simulink model "BD_CONV2"  (Simulink 4.1.1)
settings: Solver=ode1  SolverMode=SingleTasking  StartTime=0.0  StopTime=max(cyc_mph(:,1))  FixedStep=1  MaxStep=1  RelTol=1e-3  AbsTol=1e-3
undefined symbols (not defined in the file): cyc_mph, ess_on, ex_calc, fc_ct_trq, fc_emis, fc_inertia, fc_map_spd, fc_max_trq, fc_spd_scale, fc_trq_scale, fd_inertia, fd_loss, fd_ratio, gb_dnshift_load, gb_dnshift_spd, gb_gears_num, gb_inertia, gb_num_init, gb_ratio, gb_shift_delay, gb_spd_scale, gb_trq_scale, gb_upshift_load, gb_upshift_spd, logFlag, tx_eff_map, tx_map_spd, tx_map_trq, vc_clutch_bool, vc_idle_bool, vc_idle_spd, vc_key_on, vc_launch_spd, veh_air_density, veh_CD, veh_FA, veh_gravity, veh_mass, wh_axle_loss_mass, wh_axle_loss_trq, wh_front_active_bool, wh_inertia, wh_max_front_brake_force, wh_max_rear_brake_force, wh_radius, wh_rear_active_bool, wh_slip, wh_slip_force_coeff
libraries: lib_wheel2 x12, lib_drive_cycle2 x2, lib_accessory2 x2, lib_etc x2, lib_interactive x1, lib_exhaust x1, lib_fuel_converter3 x1, lib_help x1
(part 1 of 11)
settings Model: ExecutionOrder=on  LastModifiedBy=mokeefe  SaveTime=off  SaveOutput=off  LimitDataPoints=off  UnconnectedLineMsg=none  RTWTemplateMakefile=grt_vc.tmf  ExtModeTrigMode=oneshot  ExtModeArmWhenConnect=off
settings Model: ModifiedComment=|
  | mokeefe -- Thu Apr 18 07:47:12 2002 -- Version 1.98
  | saving the model:
  | o "without the model browser open"
  | o with only top-level screen visible
  | o and with "fit to view" enabled
settings Model: ModifiedHistory=|
  | mokeefe -- Thu Apr 18 07:47:12 2002 -- Version 1.98
  | saving the model:
  | o "without the model browser open"
  | o with only top-level screen visible
  | o and with "fit to view" enabled
  | 
  | mokeefe -- Thu Apr 18 07:46:46 2002 -- Version 1.97
  | saving the model:
  | o "without the model browser open"
  | o with only top-level screen visible
  | o and with "fit to view" enabled
  | 
  | mokeefe -- Thu Apr 18 07:37:24 2002 -- Version 1.96
  | saving the model
  | "without the model browser open"
  | with only top-level screen visible
  | and with "fit to view" enabled
  | 
  | abrooker -- Fri Apr 12 08:11:12 2002 -- Version 1.95
  | 
  | 
  | abrooker -- Fri Apr 12 08:02:30 2002 -- Version 1.94
  | 
  | 
  | abrooker -- Fri Apr 12 08:02:26 2002 -- Version 1.93
  | 
  | 
  | abrooker -- Fri Apr 12 07:59:19 2002 -- Version 1.92
  | 
  | 
  | abrooker -- Fri Apr 12 07:49:13 2002 -- Version 1.91
  | 
  | 
  | mokeefe -- Fri Mar 29 15:46:36 2002 -- Version 1.90
  | 
  | 
  | mokeefe -- Wed Mar 06 11:56:56 2002 -- Version 1.89
  | 
  | 
  | mokeefe -- Wed Mar 06 11:56:30 2002 -- Version 1.88
  | changed the acc_on flag in mechanical accessory loads
  | 
  | mokeefe -- Tue Mar 05 14:28:10 2002 -- Version 1.87
  | 
  | 
  | mokeefe -- Mon Mar 04 14:59:21 2002 -- Version 1.86
  | changed engine_on to key_on in Mechanical Accessory Loads <acc>
  | 
  | mokeefe -- Mon Mar 04 07:29:42 2002 -- Version 1.85
  | 
  | 
  | mokeefe -- Mon Mar 04 07:29:35 2002 -- Version 1.84
  | 
  | 
  | mokeefe -- Fri Mar 01 16:40:39 2002 -- Version 1.83
  | 
  | 
  | mokeefe -- Fri Mar 01 15:08:54 2002 -- Version 1.82
  | 
  | 
  | mokeefe -- Fri Mar 01 12:12:36 2002 -- Version 1.81
  | 
  | 
  | mokeefe -- Fri Mar 01 11:41:50 2002 -- Version 1.80
  | 
  | 
  | mokeefe -- Fri Mar 01 11:21:25 2002 -- Version 1.79
  | 
  | 
  | mokeefe -- Fri Mar 01 10:51:16 2002 -- Version 1.78
  | 
  | 
  | mokeefe -- Fri Mar 01 10:28:03 2002 -- Version 1.77
  | 
  | 
  | mokeefe -- Fri Mar 01 10:27:49 2002 -- Version 1.76
  | 
  | 
  | mokeefe -- Fri Mar 01 10:27:36 2002 -- Version 1.75
  | 
  | 
  | mokeefe -- Thu Feb 28 08:54:13 2002 -- Version 1.74
  | 
  | 
  | mokeefe -- Thu Feb 28 08:41:46 2002 -- Version 1.73
  | 
  | 
  | mokeefe -- Thu Feb 28 08:40:29 2002 -- Version 1.72
  | 
  | 
  | mokeefe -- Thu Feb 28 08:37:03 2002 -- Version 1.71
  | 
  | 
  | mokeefe -- Thu Feb 28 08:29:13 2002 -- Version 1.70
  | changing the mechanical auxiliary loads block to be more simplistic
  | 
  | mokeefe -- Wed Feb 27 14:39:18 2002 -- Version 1.69
  | 
  | 
  | mokeefe -- Wed Feb 27 14:38:57 2002 -- Version 1.68
  | 
  | 
  | mokeefe -- Wed Feb 27 14:16:01 2002 -- Version 1.67
  | changing to Mechanical Accessory Loads v2 <acc> from lib_accessory
  | 
  | mokeefe -- Wed Feb 27 14:14:56 2002 -- Version 1.66
  | 
  | 
  | mokeefe -- Tue Feb 26 10:43:51 2002 -- Version 1.65
  | changing the way that the auxiliary loads are calculated and logged to workspace. Electrical loads run on a conventional powertrain are assumed to have a mechanical to electrical efficiency penalty but are translated and added as mechanical loads
  | 
  | mokeefe -- Tue Feb 26 10:36:09 2002 -- Version 1.64
  | 
  | 
  | mokeefe -- Tue Feb 26 09:51:22 2002 -- Version 1.63
  | changed the condition for whether electrical loads are accounted in auxiliary loads block (Mechanical Accessory Loads <acc>) to be not(ess_on)
  | 
  | mokeefe -- Mon Feb 25 15:04:18 2002 -- Version 1.62
  | 
  | 
  | mokeefe -- Mon Feb 25 14:59:54 2002 -- Version 1.61
  | 
  | 
  | mokeefe -- Mon Feb 25 14:24:21 2002 -- Version 1.60
  | 
  | 
  | mokeefe -- Fri Feb 15 11:53:40 2002 -- Version 1.59
  | added and tested  Mechanical Accessory Loads <acc> block
  | 
  | mokeefe -- Thu Feb 14 17:56:13 2002 -- Version 1.58
  | 
  | 
  | mokeefe -- Thu Feb 14 17:21:52 2002 -- Version 1.57
  | 
  | 
  | mokeefe -- Thu Feb 14 17:05:06 2002 -- Version 1.56
  | updated with Mechanical Accessory Loads <acc> block
  | 
  | mokeefe -- Thu Feb 14 16:31:11 2002 -- Version 1.55
  | 
  | 
  | mokeefe -- Thu Feb 14 16:04:04 2002 -- Version 1.54
  | added Mechanical Auxiliary Loads (acc) block
  | 
  | mokeefe -- Thu Feb 14 10:48:35 2002 -- Version 1.53
  | 
  | 
  | mokeefe -- Thu Feb 14 10:41:17 2002 -- Version 1.52
  | 
  | 
  | mokeefe -- Thu Feb 14 10:24:42 2002 -- Version 1.51
  | 
  | 
  | mokeefe -- Thu Feb 14 09:59:11 2002 -- Version 1.50
  | testing
  | 
  | 
  | ssprik -- Fri Feb 09 15:14:35 2001 -- Version 1.49
  | changed foregrounds to black colors

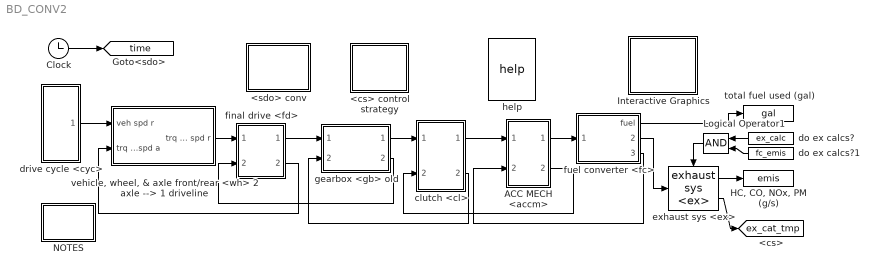
== system BD_CONV2 ==
  <cs> control strategy : Subsystem
      settings: RTWFcnNameOpts=Auto  RTWFileNameOpts=Auto
      mask Display: image(imread('bdi_cs.jpg'))
  <sdo> conv : Subsystem
      settings: RTWFcnNameOpts=Auto  RTWFileNameOpts=Auto
      mask Display: image(imread('bdi_sdo.jpg'))
  ACC MECH <accm> : Subsystem  AncestorBlock=lib_accessory2/ACC MECH <accm>  mask(Stand-Alone Mechanical Accessory Mask){generalName='acc', logPick=Log, initFileName={}, modCell={}, imgFileName='bdi_acc_pic.bmp', DEBUG=OFF}
      mask prompts: generalName "General Name of this Component [char]"; logPick "Log Variables to Workspace?"; initFileName "Initialization File(s) [cell array of char]"; modCell "Modification Cell [2 column cell array of param and val]"; imgFileName "Icon image file name [char--evaluated]"
      mask init:
      | % initialization via m-file script
      | advSACompMaskInit;
      settings: RTWFcnNameOpts=Auto  RTWFileNameOpts=Auto
      mask StyleString: edit,popup(Don't Log|Log),edit,edit,edit,popup(ON|OFF)
      mask Display: image(imread(imgFileName))
  Clock : Clock
      settings: DisplayTime=off  Decimation=10
  "HC, CO, NOx, PM (g/s)" : ToWorkspace  VariableName=emis  SampleTime=0  SaveFormat=Array
  Interactive Graphics : Subsystem  BlockChoice=off
      settings: AttributesFormatString=%<BlockChoice>  TemplateBlock=lib_interactive/Interactive Graphics  MemberBlocks=off,on  RTWFcnNameOpts=Auto  RTWFileNameOpts=Auto
  Logical Operator1 : Logic  Orientation=left  Operator=AND  Inputs=2
  NOTES : Subsystem
      settings: RTWFcnNameOpts=Auto  RTWFileNameOpts=Auto
      mask Display: disp('Version &\nCopyright')
  clutch <cl> : Subsystem  AncestorBlock=lib_transmission2/clutch <cl>  mask(Stand-Alone Clutch Mask){generalName='cl', logPick=Log, initFileName={}, modCell={}, imgFileName='bdi_cl.jpg', slip_spd=vc_launch_spd, maxtrq=max(fc_max_trq)*fc_trq_scale, DEBUG=OFF}
      mask prompts: generalName "General Name of this Component [char--evaluated]"; logPick "Log Variables to Workspace?"; initFileName "Initialization File(s) [cell array of char]"; modCell "Modification Cell [2 column cell array of param and val]"; imgFileName "Icon image file name [char--evaluated]"; slip_spd "Input shaft speed when clutch slips (rad/s):"; maxtrq "Maximum torque clutch can transmit:"
      mask help: Clutch for use with ADVISOR 2
      mask init:
      | % initialization via m-file script
      | advSACompMaskInit;
      settings: RTWFcnNameOpts=Auto  RTWFileNameOpts=Auto
      mask Help:
      | First input is req'd clutch output torque and speed, muxed together.
      | Second input is clutch state, with 1 => disengaged, 2 => slipping, and 3=> engaged.
      | Third input is available clutch input torque and limited clutch input speed.
      | First output is req'd clutch input torque and speed, muxed together.
      | Second output is available clutch output torque and limited clutch output speed.
      | The logic implemented by this block is as follows:
      |           IF (clutch is disengaged) THEN (req'd input torque=0), (req'd input speed=req'd output speed (the engine control is responsible for computing correct engine spin-down speed)), (avail. output torque=0), (limited output speed=req'd output speed)
      |           IF (clutch is slipping) THEN (req'd input torque=req'd output torque), (req'd input speed=user-defined slip speed), (avail. output torque=avail. input torque), (limited output speed=req'd output speed)
      |           IF (clutch is engaged) THEN (req'd input torque=req'd output torque), (req'd input speed=req'd output speed), (avail. output torque=avail. input torque), (limited output speed=limited input speed)
      | 
      | The clutch will transmit no more than its maximum torque as driving or braking torque.
      mask StyleString: edit,popup(Don't Log|Log),edit,edit,edit,edit,edit,popup(ON|OFF)
      mask Display: image(imread(imgFileName))
  do ex calcs? : Constant  Orientation=left  Value=ex_calc
  do ex calcs?1 : Constant  Orientation=left  Value=fc_emis
  drive cycle <cyc> : Subsystem  AncestorBlock=lib_drive_cycle2/drive cycle <cyc>  mask(Stand-Alone Drive Cycle Mask){generalName='cyc', logPick=Log, initFileName={}, modCell={}, imgFileName='bdi_cyc.jpg', DEBUG=OFF, veh_mass=veh_mass}
      mask prompts: generalName "General Name of this Component [char]"; logPick "Log Variables to Workspace?"; initFileName "Initialization File(s) [cell array of char]"; modCell "Modification Cell [2 column cell array of param and val]"; imgFileName "Icon image file name [char--evaluated]"; veh_mass "Vehicle Mass (kg)"
      mask init:
      | % initialization via m-file script
      | advSACompMaskInit;
      settings: RTWFcnNameOpts=Auto  RTWFileNameOpts=Auto
      mask StyleString: edit,popup(Don't Log|Log),edit,edit,edit,popup(ON|OFF),edit
      mask Display: image(imread(imgFileName))
  exhaust sys <ex> : lib_exhaust/exhaust sys <ex>
  final drive <fd> : Subsystem  AncestorBlock=lib_transmission2/final drive <fd>  mask(Stand-Alone Final Drive Mask){generalName='fd', logPick=Log, initFileName={}, modCell={}, imgFileName='bdi_fd.jpg', DEBUG=OFF}
      mask prompts: generalName "General Name of this Component [char]"; logPick "Log Variables to Workspace?"; initFileName "Initialization File(s) [cell array of char]"; modCell "Modification Cell [2 column cell array of param and val]"; imgFileName "Icon image file name [char--evaluated]"
      mask init:
      | % initialization via m-file script
      | advSACompMaskInit;
      settings: RTWFcnNameOpts=Auto  RTWFileNameOpts=Auto
      mask StyleString: edit,popup(Don't Log|Log),edit,edit,edit,popup(ON|OFF)
      mask Display: image(imread(imgFileName))
  fuel converter <fc> : Subsystem  AncestorBlock=lib_fuel_converter3/fuel converter <fc>  mask(Stand-Alone IC ENGINE Mask){generalName='fc', logPick=Log, initFileName={}, modCell={}, imgFileName='bdi_fc.jpg', DEBUG=OFF}
      mask prompts: generalName "General Name of this Component [char]"; logPick "Log Variables to Workspace?"; initFileName "Initialization File(s) [cell array of char]"; modCell "Modification Cell [2 column cell array of param and val]"; imgFileName "Icon image file name [char--evaluated]"
      mask init:
      | % initialization via m-file script
      | advSACompMaskInit;
      settings: RTWFcnNameOpts=Auto  RTWFileNameOpts=Auto
      mask StyleString: edit,popup(Don't Log|Log),edit,edit,edit,popup(ON|OFF)
      mask Display: image(imread(imgFileName))
  gearbox <gb> old : Subsystem  AncestorBlock=lib_transmission2/gearbox <gb> old  mask(Stand-Alone Gearbox Mask){generalName='gb', logPick=Log, initFileName={}, modCell={}, imgFileName='bdi_gb.jpg', DEBUG=OFF}
      mask prompts: generalName "General Name of this Component [char]"; logPick "Log Variables to Workspace?"; initFileName "Initialization File(s) [cell array of char]"; modCell "Modification Cell [2 column cell array of param and val]"; imgFileName "Icon image file name [char--evaluated]"
      mask init:
      | % initialization via m-file script
      | advSACompMaskInit;
      settings: RTWFcnNameOpts=Auto  RTWFileNameOpts=Auto
      mask StyleString: edit,popup(Don't Log|Log),edit,edit,edit,popup(ON|OFF)
      mask Display: image(imread(imgFileName))
  help : lib_help/help
  total fuel used (gal) : ToWorkspace  VariableName=gal  SampleTime=0  SaveFormat=Array
  "vehicle, wheel, & axle front/rear <wh> 2 axle --> 1 driveline" : Subsystem  AncestorBlock=|  mask(Stand-Alone Vehicle, Wheel, & Axle Mask){generalName='veh', generalName01='wh', logPick=Log, initFileName={}, modCell={}, imgFileName='bdi_wh&veh.jpg', DEBUG=OFF}
      | lib_wheel2/vehicle, wheel, & axle
      | front//rear <wh>
      | 2 axle --> 1 driveline
      mask prompts: generalName "General Name of Vehicle Component [char]"; generalName01 "General Name of Wheel Component [char]"; logPick "Log Variables to Workspace?"; initFileName "Initialization File(s) for VEH and WH [cell array of char]"; modCell "Modification Cell [2 column cell array of param and val]"; imgFileName "Icon image file name [char--evaluated]"
      mask init:
      | % initialization via m-file script
      | advSACompMaskInit;
      settings: RTWFcnNameOpts=Auto  RTWFileNameOpts=Auto
      mask StyleString: edit,edit,popup(Don't Log|Log),edit,edit,edit,popup(ON|OFF)
      mask Display: image(imread(imgFileName))
  tag scope: ex_cat_tmp=global, time=global
  wires:
  Clock/1 -> [time]
  final drive <fd>/1("torque and speed req'd at input side of final drive (Nm), (rad/s)") -> gearbox <gb> old/1("torque and speed req'd at output side of gearbox (Nm), (rad/s)")
  gearbox <gb> old/2("torque and speed avail. at output side of gearbox (Nm), (rad/s)") -> final drive <fd>/2("torque and speed avail. at input side of final drive (Nm), (rad/s)")
  drive cycle <cyc>/1(req'd vehicle speed (m/s)) -> "vehicle, wheel, & axle front/rear <wh> 2 axle --> 1 driveline"/1(veh spd r)
  gearbox <gb> old/1("torque and speed req'd at input side of gearbox (Nm), (rad/s)") -> clutch <cl>/1(T & w output requested)
  clutch <cl>/2(T & w output achieved) -> gearbox <gb> old/2("torque and speed avail. at input side of gearbox (Nm), (rad/s)")
  fuel converter <fc>/2(engine out emissions) -> exhaust sys <ex>/1
  fuel converter <fc>/1(fuel) -> total fuel used (gal)/1
  exhaust sys <ex>/1 -> "HC, CO, NOx, PM (g/s)"/1
  Logical Operator1/1 -> exhaust sys <ex>/Enable
  do ex calcs?/1 -> Logical Operator1/1
  do ex calcs?1/1 -> Logical Operator1/2
  exhaust sys <ex>/2 -> [ex_cat_tmp]
  clutch <cl>/1(T & w input request) -> ACC MECH <accm>/1(trq and spd out requested)
  fuel converter <fc>/3(trq and spd out achieved) -> ACC MECH <accm>/2(trq and spd in achieved)
  "vehicle, wheel, & axle front/rear <wh> 2 axle --> 1 driveline"/1(trq & spd r) -> final drive <fd>/1("torque and speed req'd at output side of final drive (Nm), (rad/s)")
  final drive <fd>/2("torque and speed avail. at output side of final drive (Nm), (rad/s)") -> "vehicle, wheel, & axle front/rear <wh> 2 axle --> 1 driveline"/2(trq & spd a)
  ACC MECH <accm>/1(trq and spd in  requested) -> fuel converter <fc>/1(trq and spd out requested)
  ACC MECH <accm>/2("trq and spd out achieved ") -> clutch <cl>/2(T & w input achieved)

== system BD_CONV2/<cs> control strategy ==
  Clutch Control : Subsystem
      settings: RTWFcnNameOpts=Auto  RTWFileNameOpts=Auto
  Drive Cycle : Subsystem
      settings: RTWFcnNameOpts=Auto  RTWFileNameOpts=Auto
  Fuel Converter Control conventional ic engine : Subsystem
      settings: RTWFcnNameOpts=Auto  RTWFileNameOpts=Auto
  Gearbox Control manual shift logic : Subsystem
      settings: RTWFcnNameOpts=Auto  RTWFileNameOpts=Auto
  Mechanical Accessories : Subsystem
      settings: RTWFcnNameOpts=Auto  RTWFileNameOpts=Auto
  Wheel Control : Subsystem
      settings: RTWFcnNameOpts=Auto  RTWFileNameOpts=Auto

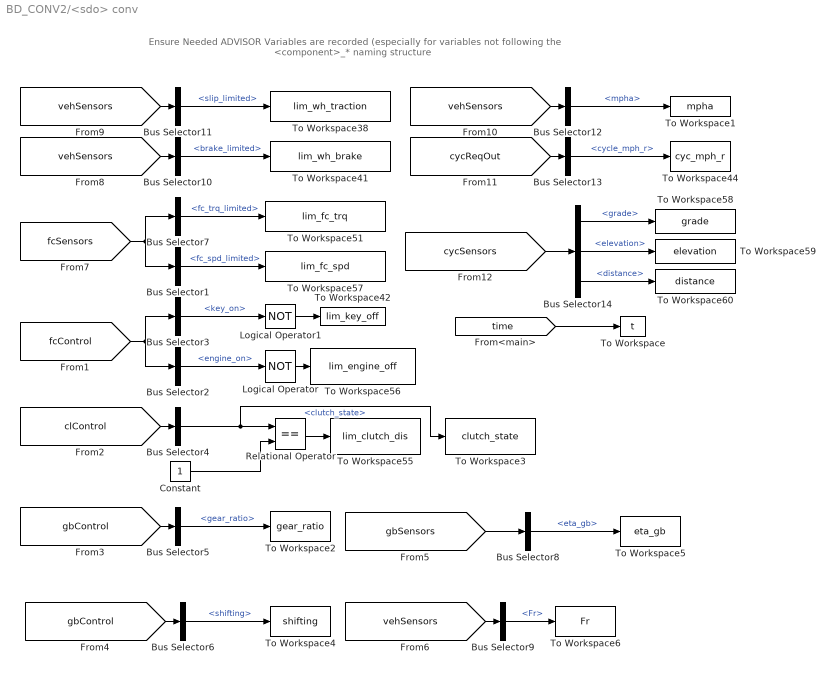
== system BD_CONV2/<sdo> conv ==
  note: Ensure Needed ADVISOR Variables are recorded
      | (especially for variables not following the <component>_* naming structure
  Bus Selector1 : BusSelector  OutputSignals=fc_spd_limited  MuxedOutput=off
  Bus Selector10 : BusSelector  OutputSignals=brake_limited  MuxedOutput=off
  Bus Selector11 : BusSelector  OutputSignals=slip_limited  MuxedOutput=off
  Bus Selector12 : BusSelector  OutputSignals=mpha  MuxedOutput=off
  Bus Selector13 : BusSelector  OutputSignals=cycle_mph_r  MuxedOutput=off
  Bus Selector14 : BusSelector  OutputSignals=grade,elevation,distance  MuxedOutput=off
  Bus Selector2 : BusSelector  OutputSignals=engine_on  MuxedOutput=off
  Bus Selector3 : BusSelector  OutputSignals=key_on  MuxedOutput=off
  Bus Selector4 : BusSelector  OutputSignals=clutch_state  MuxedOutput=off
  Bus Selector5 : BusSelector  OutputSignals=gear_ratio  MuxedOutput=off
  Bus Selector6 : BusSelector  OutputSignals=shifting  MuxedOutput=off
  Bus Selector7 : BusSelector  OutputSignals=fc_trq_limited  MuxedOutput=off
  Bus Selector8 : BusSelector  OutputSignals=eta_gb  MuxedOutput=off
  Bus Selector9 : BusSelector  OutputSignals=Fr  MuxedOutput=off
  Constant : Constant  Value=1
  Logical Operator : Logic  Operator=NOT  Inputs=1
  Logical Operator1 : Logic  Operator=NOT  Inputs=1
  Relational Operator : RelationalOperator  Operator===
  To Workspace : ToWorkspace  VariableName=t  SampleTime=0  SaveFormat=Array
  To Workspace1 : ToWorkspace  VariableName=mpha  SampleTime=-1  SaveFormat=Array
  To Workspace2 : ToWorkspace  VariableName=gear_ratio  SampleTime=-1  SaveFormat=Array
  To Workspace3 : ToWorkspace  VariableName=clutch_state  SampleTime=-1  SaveFormat=Array
  To Workspace38 : ToWorkspace  VariableName=lim_wh_traction  SampleTime=-1  SaveFormat=Array
  To Workspace4 : ToWorkspace  VariableName=shifting  SampleTime=-1  SaveFormat=Array
  To Workspace41 : ToWorkspace  VariableName=lim_wh_brake  SampleTime=-1  SaveFormat=Array
  To Workspace42 : ToWorkspace  VariableName=lim_key_off  SampleTime=-1  SaveFormat=Array
  To Workspace44 : ToWorkspace  VariableName=cyc_mph_r  SampleTime=-1  SaveFormat=Array
  To Workspace5 : ToWorkspace  VariableName=eta_gb  SampleTime=-1  SaveFormat=Array
  To Workspace51 : ToWorkspace  VariableName=lim_fc_trq  SampleTime=-1  SaveFormat=Array
  To Workspace55 : ToWorkspace  VariableName=lim_clutch_dis  SampleTime=-1  SaveFormat=Array
  To Workspace56 : ToWorkspace  VariableName=lim_engine_off  SampleTime=-1  SaveFormat=Array
  To Workspace57 : ToWorkspace  VariableName=lim_fc_spd  SampleTime=-1  SaveFormat=Array
  To Workspace58 : ToWorkspace  VariableName=grade  SampleTime=-1  SaveFormat=Array
  To Workspace59 : ToWorkspace  VariableName=elevation  SampleTime=-1  SaveFormat=Array
  To Workspace6 : ToWorkspace  VariableName=Fr  SampleTime=-1  SaveFormat=Array
  To Workspace60 : ToWorkspace  VariableName=distance  SampleTime=-1  SaveFormat=Array
  wires:
  [time] -> To Workspace/1
  Logical Operator/1 -> To Workspace56/1
  Constant/1 -> Relational Operator/2
  Relational Operator/1 -> To Workspace55/1
  Bus Selector14/3 -> To Workspace60/1  "<distance>"
  Bus Selector14/2 -> To Workspace59/1  "<elevation>"
  Bus Selector14/1 -> To Workspace58/1  "<grade>"
  Logical Operator1/1 -> To Workspace42/1
  [fcSensors] -> Bus Selector7/1, Bus Selector1/1
  Bus Selector7/1 -> To Workspace51/1  "<fc_trq_limited>"
  Bus Selector1/1 -> To Workspace57/1  "<fc_spd_limited>"
  [fcControl] -> Bus Selector3/1, Bus Selector2/1
  Bus Selector2/1 -> Logical Operator/1  "<engine_on>"
  Bus Selector3/1 -> Logical Operator1/1  "<key_on>"
  [clControl] -> Bus Selector4/1
  Bus Selector4/1 -> Relational Operator/1, To Workspace3/1  "<clutch_state>"
  [gbControl] -> Bus Selector5/1
  Bus Selector5/1 -> To Workspace2/1  "<gear_ratio>"
  [gbControl] -> Bus Selector6/1
  Bus Selector6/1 -> To Workspace4/1  "<shifting>"
  Bus Selector8/1 -> To Workspace5/1  "<eta_gb>"
  [gbSensors] -> Bus Selector8/1
  [vehSensors] -> Bus Selector9/1
  Bus Selector9/1 -> To Workspace6/1  "<Fr>"
  [vehSensors] -> Bus Selector10/1
  Bus Selector10/1 -> To Workspace41/1  "<brake_limited>"
  [vehSensors] -> Bus Selector11/1
  Bus Selector11/1 -> To Workspace38/1  "<slip_limited>"
  [vehSensors] -> Bus Selector12/1
  Bus Selector12/1 -> To Workspace1/1  "<mpha>"
  [cycReqOut] -> Bus Selector13/1
  Bus Selector13/1 -> To Workspace44/1  "<cycle_mph_r>"
  [cycSensors] -> Bus Selector14/1

== system BD_CONV2/ACC MECH <accm> ==
  note: MECHANICAL ACCESSORY
      | Interface
  trq and spd out requested : Inport  Port=1  LatchInput=off
  trq and spd in achieved : Inport  Port=2  LatchInput=off
  mechanical accessory model and interface : Subsystem  AncestorBlock=lib_accessory2/ACC MECH <accm>/mechanical accessory model and interface
      settings: RTWFcnNameOpts=Auto  RTWFileNameOpts=Auto
  trq and spd in  requested : Outport  Port=1
  "trq and spd out achieved " : Outport  Port=2
  tag scope: accReqOut=global, accSensors=global
  wires:
  mechanical accessory model and interface/4(sensors) -> [accSensors]
  [accControl] -> mechanical accessory model and interface/3(control)
  mechanical accessory model and interface/1(Out Request) -> [accReqOut]
  mechanical accessory model and interface/2(T,w in request) -> trq and spd in  requested/1
  trq and spd out requested/1 -> mechanical accessory model and interface/1("T, w out requested")
  trq and spd in achieved/1 -> mechanical accessory model and interface/2("T, w in achieved")
  mechanical accessory model and interface/3("T, w out achieved") -> "trq and spd out achieved "/1

== system BD_CONV2/Interactive Graphics ==
  off : lib_interactive/off  Tag=Altia_off  Orientation=up

== system BD_CONV2/NOTES ==
  note: ADVISOR software developed at NREL.  Copyright 1998 Midwest Research Institute.  All rights reserved.
      | Notice: These data were produced by the Midwest Research Institute (MRI) under Contract No. DE-AC98GO10337
      |      with the Department of Energy (DOE).  For a five-year period from November 6, 1998, the Government is granted for
      | itself and others acting on its behalf a nonexclusive, paid-up, irrevocable worldwide license in this data to reproduce,
      |  prepare derivative works, and perform publicly and display publicly, by or on behalf of the Government.  There is
      | provision for the possible extension of the term of this license.  Subsequent to that period or any extension granted,
      |  the Government is granted for itself and others acting on its behalf a nonexclusive, paid-up, irrevocable worldwide
  note: license in this data to reproduce, prepare derivative works, distribute copies to the public, perform publicly and display
      | publicly, and to permit others to do so.  The specific term of the license can be identified by inquiry made to the MRI
      | or DOE. Neither the United States nor the DOE, nor any of their employees, make any warranty, express or implied, or
      | assumes any legal liability or responsibility for the accuracy, completeness, or usefulness of any data, apparatus,
      | product, or process disclosed, or represents that its use would not infringe privately owned rights.
  NOTES : Subsystem
      settings: OpenFcn=advisor_ver  RTWFcnNameOpts=Auto  RTWFileNameOpts=Auto
      mask Display: disp('Double-click here or enter ''advisor_ver'' at the Matlab\ncommand line for ADVISOR version')

== system BD_CONV2/clutch <cl> ==
  note: Clutch
      | Interface
  T & w output requested : Inport  Port=1  LatchInput=off
  T & w input achieved : Inport  Port=2  LatchInput=off
  clutch model and interface : Subsystem
      settings: RTWFcnNameOpts=Auto  RTWFileNameOpts=Auto
  T & w input request : Outport  Port=1
  T & w output achieved : Outport  Port=2
  tag scope: clReqOut=global, clSensors=global
  wires:
  [clControl] -> clutch model and interface/3(control)
  clutch model and interface/1(required out) -> [clReqOut]
  clutch model and interface/4(sensors) -> [clSensors]
  clutch model and interface/3(Out2) -> T & w output achieved/1
  T & w input achieved/1 -> clutch model and interface/2(T & w input achieved)
  clutch model and interface/2(Out1) -> T & w input request/1
  T & w output requested/1 -> clutch model and interface/1(T & w output requested)

== system BD_CONV2/drive cycle <cyc> ==
  note: DRIVE CYCLE
  drive cycle model and interface : lib_drive_cycle2/drive cycle <cyc>/drive cycle model and interface
      settings: RTWFcnNameOpts=Auto  RTWFileNameOpts=Auto
  req'd vehicle speed (m/s) : Outport  Port=1  InitialOutput=0
  tag scope: cycReqOut=global, cycSensors=global
  wires:
  drive cycle model and interface/2 -> req'd vehicle speed (m/s)/1
  [cycControl] -> drive cycle model and interface/1
  drive cycle model and interface/1 -> [cycReqOut]
  drive cycle model and interface/3 -> [cycSensors]

== system BD_CONV2/final drive <fd> ==
  "torque and speed req'd at output side of final drive (Nm), (rad/s)" : Inport  Port=1  LatchInput=off
  "torque and speed avail. at input side of final drive (Nm), (rad/s)" : Inport  Port=2  LatchInput=off
  Block NOTES : Subsystem
      settings: RTWFcnNameOpts=Auto  RTWFileNameOpts=Auto
      mask Display: disp('Block\nNOTES')
  final drive model & interface : Subsystem
      settings: RTWFcnNameOpts=Auto  RTWFileNameOpts=Auto
  help : Subsystem
      settings: OpenFcn=web(['file:\\\' which('wheel_axle.htm')]);  RTWFcnNameOpts=Auto  RTWFileNameOpts=Auto
      mask Display: image(imread('doc_man.jpg'))
  "torque and speed req'd at input side of final drive (Nm), (rad/s)" : Outport  Port=1  InitialOutput=0
  "torque and speed avail. at output side of final drive (Nm), (rad/s)" : Outport  Port=2  InitialOutput=0
  tag scope: fdReqOut=global, fdSensors=global
  wires:
  final drive model & interface/3(T & w output achieved) -> "torque and speed avail. at output side of final drive (Nm), (rad/s)"/1
  final drive model & interface/2(T & w input request) -> "torque and speed req'd at input side of final drive (Nm), (rad/s)"/1
  "torque and speed avail. at input side of final drive (Nm), (rad/s)"/1 -> final drive model & interface/2(T & w input achieved)
  "torque and speed req'd at output side of final drive (Nm), (rad/s)"/1 -> final drive model & interface/1(T & w output request)
  final drive model & interface/4(sensors) -> [fdSensors]
  [fdControl] -> final drive model & interface/3(control)
  final drive model & interface/1(out request) -> [fdReqOut]

== system BD_CONV2/fuel converter <fc> ==
  note: Internal Combustion Engine
  trq and spd out requested : Inport  Port=1  LatchInput=off
  Block NOTES : Subsystem
      settings: RTWFcnNameOpts=Auto  RTWFileNameOpts=Auto
      mask Display: disp('Block\nNOTES')
  IC Engine Model  &  Interface : Subsystem
      settings: RTWFcnNameOpts=Auto  RTWFileNameOpts=Auto
  help : Subsystem
      settings: OpenFcn=web(['file:\\\' which('fuel_converter.htm')]);  RTWFcnNameOpts=Auto  RTWFileNameOpts=Auto
      mask Display: image(imread('doc_man.jpg'))
  fuel : Outport  Port=1
  engine out emissions : Outport  Port=2
  trq and spd out achieved : Outport  Port=3
  tag scope: fcReqOut=global, fcSensors=global
  wires:
  IC Engine Model  &  Interface/1(req out) -> [fcReqOut]
  IC Engine Model  &  Interface/2(fuel) -> fuel/1
  IC Engine Model  &  Interface/3(engine out emissions) -> engine out emissions/1
  IC Engine Model  &  Interface/4(trq and spd out achieved) -> trq and spd out achieved/1
  IC Engine Model  &  Interface/5(sensors) -> [fcSensors]
  [fcControl] -> IC Engine Model  &  Interface/2(control)
  trq and spd out requested/1 -> IC Engine Model  &  Interface/1(trq and spd out requested)

== system BD_CONV2/gearbox <gb> old ==
  note: Gearbox
  "torque and speed req'd at output side of gearbox (Nm), (rad/s)" : Inport  Port=1  LatchInput=off
  "torque and speed avail. at input side of gearbox (Nm), (rad/s)" : Inport  Port=2  LatchInput=off
  Block NOTES : Subsystem
      settings: RTWFcnNameOpts=Auto  RTWFileNameOpts=Auto
      mask Display: disp('Block\nNOTES')
  gearbox model & interface : Subsystem
      settings: RTWFcnNameOpts=Auto  RTWFileNameOpts=Auto
  help : Subsystem
      settings: OpenFcn=web(['file:\\\' which('gearbox.htm')]);  RTWFcnNameOpts=Auto  RTWFileNameOpts=Auto
      mask Display: image(imread('doc_man.jpg'))
  "torque and speed req'd at input side of gearbox (Nm), (rad/s)" : Outport  Port=1  InitialOutput=0
  "torque and speed avail. at output side of gearbox (Nm), (rad/s)" : Outport  Port=2  InitialOutput=0
  tag scope: gbReqOut=global, gbSensors=global
  wires:
  gearbox model & interface/4(sensors) -> [gbSensors]
  [gbControl] -> gearbox model & interface/3(controls)
  gearbox model & interface/3(trq and spd output achieved) -> "torque and speed avail. at output side of gearbox (Nm), (rad/s)"/1
  "torque and speed avail. at input side of gearbox (Nm), (rad/s)"/1 -> gearbox model & interface/2(trq and spd input achieved)
  "torque and speed req'd at output side of gearbox (Nm), (rad/s)"/1 -> gearbox model & interface/1(trq and spd output request)
  gearbox model & interface/2(trq and spd input request) -> "torque and speed req'd at input side of gearbox (Nm), (rad/s)"/1
  gearbox model & interface/1(requested output) -> [gbReqOut]

== system BD_CONV2/vehicle, wheel, & axle front/rear <wh> 2 axle --> 1 driveline ==
  note: Vehicle, Wheel, and Axle
      | 2 axles --> 1 driveline
  veh spd r : Inport  Port=1  LatchInput=off
  trq & spd a : Inport  Port=2  LatchInput=off
  models and interface : Subsystem  AncestorBlock=|
      | lib_wheel2/vehicle, wheel, & axle
      | front//rear <wh>
      | 2 axle --> 1 driveline/models and interface
      settings: RTWFcnNameOpts=Auto  RTWFileNameOpts=Auto
  trq & spd r : Outport  Port=1  InitialOutput=0
  tag scope: vehReqOut=global, vehSensors=global
  wires:
  veh spd r/1 -> models and interface/1(vehicle speed req'd at end of time step (m/s))
  trq & spd a/1 -> models and interface/2("torque and speed available from drivetrain into axles (Nm), (rad/s)")
  [vehControl] -> models and interface/3(control)
  models and interface/1(requested out) -> [vehReqOut]
  models and interface/2(torque and speed req'd from drivetrain into axles (Nm),(rad/s)) -> trq & spd r/1
  models and interface/3(sensors) -> [vehSensors]

== system BD_CONV2/<cs> control strategy/Clutch Control ==
  Bus Creator : BusCreator  Inputs=3
  Bus Selector : BusSelector  OutputSignals=mpha  MuxedOutput=off
  Bus Selector1 : BusSelector  OutputSignals=shifting  MuxedOutput=off
  Bus Selector2 : BusSelector  OutputSignals=gb_spd_in_a  MuxedOutput=off
  Bus Selector3 : BusSelector  OutputSignals=clutch_trq_out_r  MuxedOutput=off
  Bus Selector4 : BusSelector  OutputSignals=clutch_spd_out_r  MuxedOutput=off
  Bus Selector5 : BusSelector  OutputSignals=veh_spd_a_rec  MuxedOutput=off
  Bus Selector6 : BusSelector  OutputSignals=cycle_mph_r  MuxedOutput=off
  Bus Selector7 : BusSelector  OutputSignals=v_ave_req  MuxedOutput=off
  Clutch Control : Subsystem  TreatAsAtomicUnit=on
      settings: RTWFcnNameOpts=Auto  RTWFileNameOpts=Auto
  Memory1 : Memory  X0=0  InheritSampleTime=off
      settings: RTWStateStorageClass=Auto
  Memory2 : Memory  X0=cyc_mph(1,2)  InheritSampleTime=off
      settings: RTWStateStorageClass=Auto
  Memory3 : Memory  X0=0  InheritSampleTime=off
      settings: RTWStateStorageClass=Auto
  Memory4 : Memory  X0=cyc_mph(1,2)  InheritSampleTime=off
      settings: RTWStateStorageClass=Auto
  tag scope: clControl=global
  wires:
  Memory4/1 -> Clutch Control/7(cyc_mph_r)
  Memory3/1 -> Clutch Control/6(veh_spd_a_rec)
  Memory2/1 -> Clutch Control/5(mpha)
  Memory1/1 -> Clutch Control/2(gb_spd_in_a)
  Clutch Control/3(launch_flag) -> Bus Creator/3  "launch_flag"
  Bus Selector4/1 -> Clutch Control/4(w_cl_out)  "<clutch_spd_out_r>"
  Bus Selector3/1 -> Clutch Control/3(T_cl_out)  "<clutch_trq_out_r>"
  [clReqOut] -> Bus Selector4/1, Bus Selector3/1
  Bus Selector2/1 -> Memory1/1  "<gb_spd_in_a>"
  [gbSensors] -> Bus Selector2/1
  Bus Selector1/1 -> Clutch Control/1(shifting)  "<shifting>"
  [gbControl] -> Bus Selector1/1
  Clutch Control/2(launch_speed) -> Bus Creator/2  "launch_speed"
  Clutch Control/1(clutch_state) -> Bus Creator/1  "clutch_state"
  Bus Creator/1 -> [clControl]
  [vehSensors] -> Bus Selector/1
  Bus Selector/1 -> Memory2/1  "<mpha>"
  [vehSensors] -> Bus Selector5/1
  Bus Selector5/1 -> Memory3/1  "<veh_spd_a_rec>"
  [cycReqOut] -> Bus Selector6/1
  Bus Selector6/1 -> Memory4/1  "<cycle_mph_r>"
  [vehReqOut] -> Bus Selector7/1
  Bus Selector7/1 -> Clutch Control/8(v_ave_req)  "<v_ave_req>"

== system BD_CONV2/<cs> control strategy/Drive Cycle ==
  Bus Creator : BusCreator  Inputs=4
  Bus Selector : BusSelector  OutputSignals=mpha  MuxedOutput=off
  Constant : Constant  Value=0
  drive cycle dummy controller : lib_drive_cycle2/drive cycle controls/drive cycle dummy controller
      settings: RTWFcnNameOpts=Auto  RTWFileNameOpts=Auto
  tag scope: cycControl=global
  wires:
  [vehSensors] -> Bus Selector/1
  Bus Selector/1 -> drive cycle dummy controller/1  "<mpha>"
  Constant/1 -> drive cycle dummy controller/3, drive cycle dummy controller/2, drive cycle dummy controller/4
  drive cycle dummy controller/1 -> Bus Creator/1  "mpha"
  drive cycle dummy controller/2 -> Bus Creator/2  "altia_grade"
  drive cycle dummy controller/3 -> Bus Creator/3  "Altia_Run"
  drive cycle dummy controller/4 -> Bus Creator/4  "altia_cyc_mph_r"
  Bus Creator/1 -> [cycControl]

== system BD_CONV2/<cs> control strategy/Fuel Converter Control conventional ic engine ==
  conventional IC engine : Subsystem
      settings: RTWFcnNameOpts=Auto  RTWFileNameOpts=Auto

== system BD_CONV2/<cs> control strategy/Gearbox Control manual shift logic ==
  Bus Selector : BusSelector  OutputSignals=acc_mech_trq_a  MuxedOutput=off
  Bus Selector1 : BusSelector  OutputSignals=mpha  MuxedOutput=off
  Bus Selector10 : BusSelector  OutputSignals=eta_gb  MuxedOutput=off
  Bus Selector2 : BusSelector  OutputSignals=cycle_mph_r  MuxedOutput=off
  Bus Selector3 : BusSelector  OutputSignals=veh_spd_a_rec  MuxedOutput=off
  Bus Selector4 : BusSelector  OutputSignals=slip_limited  MuxedOutput=off
  Bus Selector7 : BusSelector  OutputSignals=gb_trq_out_r  MuxedOutput=off
  Bus Selector8 : BusSelector  OutputSignals=gb_spd_out_r  MuxedOutput=off
  Bus Selector9 : BusSelector  OutputSignals=gb_spd_in_a  MuxedOutput=off
  Memory{,1,3,5} (4 alike) : Memory  X0=0  InheritSampleTime=off
      settings: RTWStateStorageClass=Auto
  Memory2 : Memory  X0=cyc_mph(1,2)  InheritSampleTime=off
      settings: RTWStateStorageClass=Auto
  Memory4 : Memory  X0=cyc_mph(1,2)  InheritSampleTime=off
      settings: RTWStateStorageClass=Auto
  Mux1 : Mux  Inputs=3
  manual shift logic : Subsystem  TreatAsAtomicUnit=on
      settings: RTWFcnNameOpts=Auto  RTWFileNameOpts=Auto
  tag scope: gbControl=global
  wires:
  Memory4/1 -> manual shift logic/7("cyc_mph_r, t=(i-1)")
  Memory3/1 -> manual shift logic/8("veh_spd_a_rec, t=(i-1)")
  Memory2/1 -> manual shift logic/6("mpha, t=(i-1)")
  Memory1/1 -> manual shift logic/2("gb_spd_in_a, t=(i-1)")
  Memory/1 -> manual shift logic/1("eta_gb, t=(i-1)")
  [gbReqOut] -> Bus Selector7/1, Bus Selector8/1
  Bus Selector7/1 -> manual shift logic/4(T_gb_out)  "<gb_trq_out_r>"
  Bus Selector8/1 -> manual shift logic/3(w_gb_out)  "<gb_spd_out_r>"
  Bus Selector9/1 -> Memory1/1  "<gb_spd_in_a>"
  Bus Selector10/1 -> Memory/1  "<eta_gb>"
  [gbSensors] -> Bus Selector9/1, Bus Selector10/1
  Mux1/1 -> [gbControl]
  manual shift logic/3(gear number) -> Mux1/3  "gear_number"
  manual shift logic/2(shifting) -> Mux1/2  "shifting"
  manual shift logic/1(gear ratio) -> Mux1/1  "gear_ratio"
  [accSensors] -> Bus Selector/1
  Bus Selector/1 -> Memory5/1  "<acc_mech_trq_a>"
  Memory5/1 -> manual shift logic/5(acc_mech_trq_est)
  [vehSensors] -> Bus Selector1/1
  Bus Selector1/1 -> Memory2/1  "<mpha>"
  [cycReqOut] -> Bus Selector2/1
  Bus Selector2/1 -> Memory4/1  "<cycle_mph_r>"
  [vehSensors] -> Bus Selector3/1
  Bus Selector3/1 -> Memory3/1  "<veh_spd_a_rec>"
  [vehReqOut] -> Bus Selector4/1
  Bus Selector4/1 -> manual shift logic/9(slip_limited)  "<slip_limited>"

== system BD_CONV2/<cs> control strategy/Mechanical Accessories ==
  Bus Creator : BusCreator  Inputs=9
  Bus Selector : BusSelector  OutputSignals=fc_spd_est  MuxedOutput=off
  Bus Selector1 : BusSelector  OutputSignals=F_req  MuxedOutput=off
  Bus Selector2 : BusSelector  OutputSignals=key_on  MuxedOutput=off
  Bus Selector3 : BusSelector  OutputSignals=engine_on  MuxedOutput=off
  Constant : Constant  Value=not(ess_on)*1
  Constant1 : Constant  Value=inf
  Constant2 : Constant  Value=(vc_idle_spd*vc_idle_bool)+eps
  mechanical accessory controller : Subsystem
      settings: RTWFcnNameOpts=Auto  RTWFileNameOpts=Auto
  tag scope: accControl=global
  wires:
  Constant1/1 -> mechanical accessory controller/2(maximum accessory speed)
  Constant2/1 -> mechanical accessory controller/3(minimum accessory speed)
  Constant/1 -> mechanical accessory controller/4(electrical accessories on?)
  mechanical accessory controller/1(acc_on) -> Bus Creator/1
  mechanical accessory controller/2(acc_mech_spd_r) -> Bus Creator/2
  mechanical accessory controller/3(acc_mech_spd_a) -> Bus Creator/3
  mechanical accessory controller/4(acc_max_spd) -> Bus Creator/4
  mechanical accessory controller/5(acc_min_spd) -> Bus Creator/5
  mechanical accessory controller/6(elec_acc_on_bool) -> Bus Creator/6
  mechanical accessory controller/7(F_req) -> Bus Creator/7
  mechanical accessory controller/8(key_on) -> Bus Creator/8
  mechanical accessory controller/9(engine_on) -> Bus Creator/9
  Bus Creator/1 -> [accControl]
  [fcControl] -> Bus Selector2/1
  Bus Selector2/1 -> mechanical accessory controller/6(key on?)  "<key_on>"
  [fcControl] -> Bus Selector3/1
  Bus Selector3/1 -> mechanical accessory controller/7(engine on?)  "<engine_on>"
  [fcReqOut] -> Bus Selector/1
  Bus Selector/1 -> mechanical accessory controller/1(accessory reference shaft speed)  "<fc_spd_est>"
  [vehReqOut] -> Bus Selector1/1
  Bus Selector1/1 -> mechanical accessory controller/5(Force required for vehicle motion)  "<F_req>"

== system BD_CONV2/<cs> control strategy/Wheel Control ==
  Bus Selector : BusSelector  OutputSignals=v_init  MuxedOutput=off
  Bus Selector1 : BusSelector  OutputSignals=current_veh_mass  MuxedOutput=off
  Bus Selector2 : BusSelector  OutputSignals=grade  MuxedOutput=off
  dummy controls : lib_wheel2/vehicle controls/dummy controls
      settings: RTWFcnNameOpts=Auto  RTWFileNameOpts=Auto
  tag scope: vehControl=global
  wires:
  [cycReqOut] -> Bus Selector/1
  Bus Selector/1 -> dummy controls/1  "<v_init>"
  Bus Selector1/1 -> dummy controls/2  "<current_veh_mass>"
  Bus Selector2/1 -> dummy controls/3  "<grade>"
  [cycSensors] -> Bus Selector2/1
  [cycSensors] -> Bus Selector1/1
  dummy controls/1 -> [vehControl]

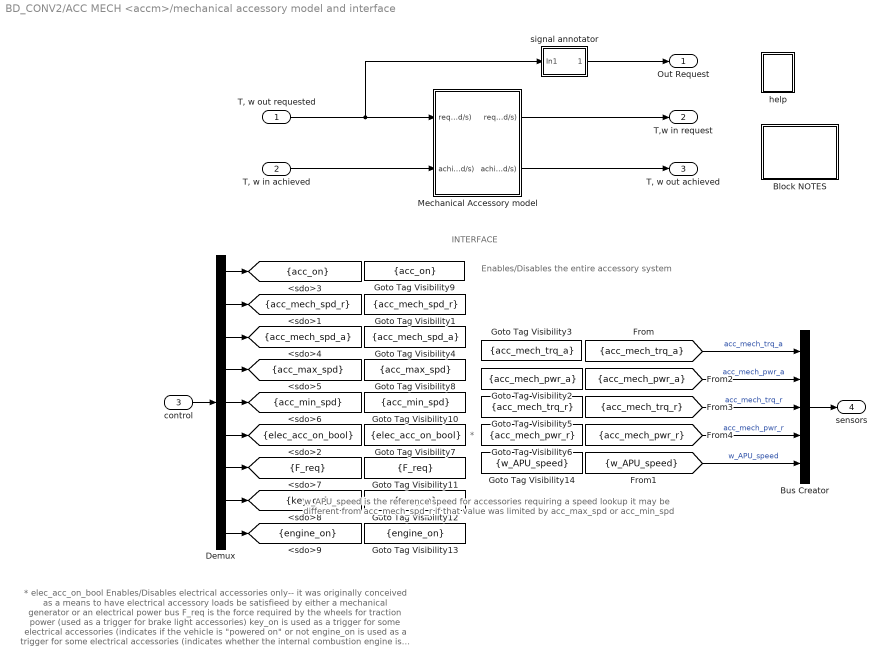
== system BD_CONV2/ACC MECH <accm>/mechanical accessory model and interface ==
  note: w_APU_speed is the reference speed for accessories requiring a speed lookup
      | it may be different from acc_mech_spd_r if that value was limited by acc_max_spd
      | or acc_min_spd
  note: * elec_acc_on_bool Enables/Disables electrical accessories only-- it was originally conceived as a means to have electrical accessory loads be
      | satisfieed by either a mechanical generator or an electrical power bus
      |
      | F_req is the force required by the wheels for traction power (used as a trigger for brake light accessories)
      |
      | key_on is used as a trigger for some electrical accessories (indicates if the vehicle is "powered on" or not
      |
      | engine_on is used as a trigger for some electrical accessories (indicates whether the internal combustion engine is running or not) used
      | for starter motor
  note: *
  note: Enables/Disables the entire accessory system
  note: INTERFACE
  "T, w out requested" : Inport  Port=1  LatchInput=off
  "T, w in achieved" : Inport  Port=2  LatchInput=off
  control : Inport  Port=3  LatchInput=off
  Block NOTES : Subsystem
      settings: RTWFcnNameOpts=Auto  RTWFileNameOpts=Auto
      mask Display: disp('Block\nNOTES')
  Bus Creator : BusCreator  Inputs=5
  Demux : Demux  Outputs=9  BusSelectionMode=off
  Goto Tag Visibility1 : GotoTagVisibility  GotoTag=acc_mech_spd_r
  Goto Tag Visibility10 : GotoTagVisibility  GotoTag=acc_min_spd
  Goto Tag Visibility11 : GotoTagVisibility  GotoTag=F_req
  Goto Tag Visibility12 : GotoTagVisibility  GotoTag=key_on
  Goto Tag Visibility13 : GotoTagVisibility  GotoTag=engine_on
  Goto Tag Visibility14 : GotoTagVisibility  GotoTag=w_APU_speed
  Goto Tag Visibility2 : GotoTagVisibility  GotoTag=acc_mech_pwr_a
  Goto Tag Visibility3 : GotoTagVisibility  GotoTag=acc_mech_trq_a
  Goto Tag Visibility4 : GotoTagVisibility  GotoTag=acc_mech_spd_a
  Goto Tag Visibility5 : GotoTagVisibility  GotoTag=acc_mech_trq_r
  Goto Tag Visibility6 : GotoTagVisibility  GotoTag=acc_mech_pwr_r
  Goto Tag Visibility7 : GotoTagVisibility  GotoTag=elec_acc_on_bool
  Goto Tag Visibility8 : GotoTagVisibility  GotoTag=acc_max_spd
  Goto Tag Visibility9 : GotoTagVisibility  GotoTag=acc_on
  Mechanical Accessory model : Subsystem
      settings: RTWFcnNameOpts=Auto  RTWFileNameOpts=Auto
      mask Display: image(imread('bdi_acc_pic.bmp'))
  help : Subsystem
      settings: OpenFcn=web(['file:\\\' which('motor_controller.htm')]);  RTWFcnNameOpts=Auto  RTWFileNameOpts=Auto
      mask Display: image(imread('doc_man.jpg'))
  signal annotator : Subsystem
      settings: RTWFcnNameOpts=Auto  RTWFileNameOpts=Auto
  Out Request : Outport  Port=1
  T,w in request : Outport  Port=2
  "T, w out achieved" : Outport  Port=3
  sensors : Outport  Port=4
  tag scope: F_req=scoped, acc_max_spd=scoped, acc_mech_spd_a=scoped, acc_mech_spd_r=scoped, acc_min_spd=scoped, acc_on=scoped, elec_acc_on_bool=scoped, engine_on=scoped, key_on=scoped
  wires:
  Demux/9 -> [engine_on]
  Demux/8 -> [key_on]
  Demux/7 -> [F_req]
  [w_APU_speed] -> Bus Creator/5  "w_APU_speed"
  Demux/6 -> [elec_acc_on_bool]
  signal annotator/1(Out1) -> Out Request/1
  control/1 -> Demux/1
  Bus Creator/1 -> sensors/1
  Demux/5 -> [acc_min_spd]
  Demux/4 -> [acc_max_spd]
  Demux/3 -> [acc_mech_spd_a]
  [acc_mech_pwr_r] -> Bus Creator/4  "acc_mech_pwr_r"
  [acc_mech_trq_r] -> Bus Creator/3  "acc_mech_trq_r"
  [acc_mech_pwr_a] -> Bus Creator/2  "acc_mech_pwr_a"
  [acc_mech_trq_a] -> Bus Creator/1  "acc_mech_trq_a"
  Demux/2 -> [acc_mech_spd_r]
  Demux/1 -> [acc_on]
  Mechanical Accessory model/2("achieved shaft T and w, out to the driveline (Nm ; rad/s)") -> "T, w out achieved"/1
  "T, w in achieved"/1 -> Mechanical Accessory model/2("achieved shaft and belt T and w, in from the prime mover (Nm ; rad/s)")
  Mechanical Accessory model/1("requested shaft and belt T and w, in from the prime mover (Nm ; rad/s)") -> T,w in request/1
  "T, w out requested"/1 -> signal annotator/1(In1), Mechanical Accessory model/1("requested shaft T and w, out to the driveline  (Nm ; rad/s; rad/s)")

== system BD_CONV2/NOTES/NOTES ==
  note: ADVISOR 2.0.2 10/7/98
      | Copyright 1998-2003  MRI, NREL.
      | All rights reserved
      |
      |  Notice:  This computer software was
      |  prepared by NREL/MRI, and hereinafter the Contractor,
      | under Contract No. DE-AC36-83CH10093 with
      | the Department of Energy (DOE).  All rights
      | in the computer software are reserved by DOE
      | on behalf of the United States Government and
      | the Contractor as provided in the contract.
      | You are authorized to use this computer software
      | for Governmental purposes but it is not to be
      | released or distributed to the public.  NEITHER
      | THE GOVERNMENT NOR THE CONTRACTOR MAKES ANY
      | WARRANTY, EXPRESS OR IMPLIED, OR ASSUMES ANY
      | LIABILITY FOR THE USE OF THIS SOFTWARE.
      | This notice including this sentence must
      | appear on any copies of this computer software.

== system BD_CONV2/clutch <cl>/clutch model and interface ==
  note: Model
  note: Interface
  T & w output requested : Inport  Port=1  LatchInput=off
  T & w input achieved : Inport  Port=2  LatchInput=off
  control : Inport  Port=3  LatchInput=off
  Demux2 : Demux  Outputs=3  BusSelectionMode=off
  Goto Tag Visibility : GotoTagVisibility  GotoTag=clutch_state
  Goto Tag Visibility1 : GotoTagVisibility  GotoTag=T_cl_out
  Goto Tag Visibility2 : GotoTagVisibility  GotoTag=w_cl_out
  Goto Tag Visibility3 : GotoTagVisibility  GotoTag=launch_speed
  Goto Tag Visibility4 : GotoTagVisibility  GotoTag=launch_flag
  Mux2 : Mux  Inputs=2
  clutch model : Subsystem
      settings: RTWFcnNameOpts=Auto  RTWFileNameOpts=Auto
  signal annotator : Subsystem
      settings: RTWFcnNameOpts=Auto  RTWFileNameOpts=Auto
  required out : Outport  Port=1
  Out1 : Outport  Port=2
  Out2 : Outport  Port=3
  sensors : Outport  Port=4
  tag scope: clutch_state=scoped, launch_flag=scoped, launch_speed=scoped
  wires:
  signal annotator/1(Out1) -> required out/1
  Mux2/1 -> sensors/1
  clutch model/2(T & w output achieved) -> Out2/1
  T & w input achieved/1 -> clutch model/2(T & w input achieved)
  clutch model/1(T & w input request) -> Out1/1
  T & w output requested/1 -> signal annotator/1(In1), clutch model/1(T & w output requested)
  [w_cl_out] -> Mux2/2
  [T_cl_out] -> Mux2/1
  Demux2/3 -> [launch_flag]
  Demux2/2 -> [launch_speed]
  Demux2/1 -> [clutch_state]
  control/1 -> Demux2/1

== system BD_CONV2/final drive <fd>/Block NOTES ==
  note: The inertia torque is the input torque required to accelerate the
      | final drive's inertia as measured on the input side.
  note: The loss torque is zero when the gears are not turning,
      | and is applied at the input side of the gear reduction.
  note: This final drive model includes loss data, rotational inertia, and a gear reduction.

== system BD_CONV2/final drive <fd>/final drive model & interface ==
  note: Model
  note: Interface
  T & w output request : Inport  Port=1  LatchInput=off
  T & w input achieved : Inport  Port=2  LatchInput=off
  control : Inport  Port=3  LatchInput=off
  Ground : Ground
  Terminator : Terminator
  final drive model : Subsystem
      settings: RTWFcnNameOpts=Auto  RTWFileNameOpts=Auto
  signal annotator : Subsystem
      settings: RTWFcnNameOpts=Auto  RTWFileNameOpts=Auto
  out request : Outport  Port=1  InitialOutput=0
  T & w input request : Outport  Port=2  InitialOutput=0
  T & w output achieved : Outport  Port=3  InitialOutput=0
  sensors : Outport  Port=4  InitialOutput=0
  wires:
  signal annotator/1(Out1) -> out request/1
  control/1 -> Terminator/1
  Ground/1 -> sensors/1
  final drive model/2("torque and speed avail. at output side of final drive (Nm), (rad/s)") -> T & w output achieved/1
  T & w input achieved/1 -> final drive model/2("torque and speed avail. at input side of final drive (Nm), (rad/s)")
  T & w output request/1 -> signal annotator/1(In1), final drive model/1("torque and speed req'd at output side of final drive (Nm), (rad/s)")
  final drive model/1("torque and speed req'd at input side of final drive (Nm), (rad/s)") -> T & w input request/1

== system BD_CONV2/final drive <fd>/help ==

== system BD_CONV2/fuel converter <fc>/Block NOTES ==
  note: This block models the internal combustion engine, and includes inertia effects,
      | performance limits, accessory loads, and temperature transient effects on fuel
      | use, engine-out emissions, and catalyst efficiency.  There are 'leads' to the
      | engine controller here, which controller determines whether the engine is on.
